simulink model "EcoSIM3_P2_C2_WIP"  (R2014b)
settings: Solver=ode1  SolverMode=SingleTasking  StartTime=0.0  StopTime=4  FixedStep=0.01  RelTol=1e-3
PostLoadFcn:
  | %, if any(exist('dsrtsu_mdlpostloadfcn', 'file') == [2, 3, 6]), try dsrtsu_mdlpostloadfcn('Execute', bdroot); catch fprintf('Error in PostLoadFcn (dsrtsu_mdlpostloadfcn) for model "%s":\n %s\n', bdroot, lasterr); end, end,
InitFcn:
  | tic
  | %Startup_EcoSIM
undefined symbols (not defined in the file or in its folder): canChannel, Controls, DriveCycles, Driver, EM_EFF_MAP, EM_PwrLoss_MAP, EngPwr, EngSpd, EngTrq, Glbl, Overwritten_Mode, Plants, Power, sigbuilder_block, Torque, Trialmap, Veh_Dynamics
libraries: simulink x135, canmsglib x113, fl_lib x104, canlib x89, nesl_utility x56, sdl_lib x29, dspsigops x6, dspswit3 x5, dspstat3 x2, commnoisgen2 x1, dspfdesign x1
(part 16 of 21)

== system EcoSIM3_P2_C2_WIP/Powertrain/Clutch_Transmission2/Trans_Plant/Plant/Subsystem/Lookup Table based Gear ==
  y12 : Inport
  y34 : Inport  Port=2
  y5R : Inport  Port=3
  Bias : Bias  Bias=-1
  Bias1 : Bias  Bias=-1
  Bias2 : Bias  Bias=-1
  Direct Lookup Table (n-D) : LookupNDDirect  NumberOfTableDimensions=3  Table=cat(3,[8 8 8; 8 5 8; 8 8 8], [8 1 8; 3 0 4; 8 2 8],[8 8 8; 8 -1 8; 8 8 8])
  Gear : Outport
  wires:
  Bias/1 -> Direct Lookup Table (n-D)/1
  Bias1/1 -> Direct Lookup Table (n-D)/2
  Bias2/1 -> Direct Lookup Table (n-D)/3
  y12/1 -> Bias/1
  Direct Lookup Table (n-D)/1 -> Gear/1
  y5R/1 -> Bias2/1
  y34/1 -> Bias1/1

== system EcoSIM3_P2_C2_WIP/Powertrain/Electric Motor / Component Model/Plant/EM_Thermal_Model/EM_Over_Temp_Fault ==
  In1 : Inport
  Bus Selector : BusSelector  OutputSignals=Temp_deg_C,EM_OverTemp_Trigger
  Switch : Switch  Criteria=u2 > Threshold  Threshold=0.5
  Out1 : Outport
  wires:
  [EM_Over_temperature_Trigger] -> Bus Selector/1
  Bus Selector/1 -> Switch/1  "<Temp_deg_C>"
  Bus Selector/2 -> Switch/2  "<EM_OverTemp_Trigger>"
  Switch/1 -> Out1/1
  In1/1 -> Switch/3

== system EcoSIM3_P2_C2_WIP/Powertrain/Electric Motor / Component Model/Plant/EM_Thermal_Model/Heat Dissipated through coolant ==
  Coolant Out Temp : Inport
  Add1 : Sum  Inputs=+-
  Coolant Heat Capacity : Gain  Gain=3148
  Coolant Flow rate lit/min : Constant  Value=4
  Coolant Inlet Temp (K) : Constant  Value=293
  Product : Product
  Simulink-PS Converter2 : nesl_utility/Simulink-PS Converter  PhysicalDomain=network_engine_domain  SubClassName=ps_input  LeftPortType=input  RightPortType=output  PseudoPeriodic=off  Frequencies=[]  NoiseDistribution=none  NoiseParameters=[]  Unit=J/s  AffineConversion=off  InputFiltering=off  SimscapeFilterOrder=1  InputFilterTimeConstant=0.001  UdotUserProvided=1
  Subtract : Gain  Gain=-1
  per sec : Gain  Gain=1/60
  Coolant Heat Gain : PMIOPort  Port=1  Side=Right
  wires:
  Product/1 -> Subtract/1  "EM_Coolant_Heat_Reject_W"
  Coolant Heat Capacity/1 -> Product/2
  Add1/1 -> Product/1
  Coolant Inlet Temp (K)/1 -> Add1/2
  Subtract/1 -> Simulink-PS Converter2/1
  Coolant Out Temp/1 -> Add1/1
  per sec/1 -> Coolant Heat Capacity/1
  Coolant Flow rate lit/min/1 -> per sec/1
  connections:
  Simulink-PS Converter2/RConn1 -- Coolant Heat Gain/RConn1

== system EcoSIM3_P2_C2_WIP/Powertrain/Electric Motor / Component Model/Plant/EM_Thermal_Model/Temp Hotspot ==
  Add1 : Sum  Inputs=+-
  Constant3 : Constant  Value=273
  Ideal Temperature Sensor1 : fl_lib/Thermal/Thermal Sensors/Ideal Temperature Sensor
  PS-Simulink Converter1 : nesl_utility/PS-Simulink Converter  PhysicalDomain=network_engine_domain  SubClassName=ps_output  LeftPortType=input  RightPortType=output  PseudoPeriodic=off  Frequencies=[]  Unit=K  AffineConversion=off
  Thermal Reference5 : fl_lib/Thermal/Thermal Elements/Thermal Reference
  Conn1 : PMIOPort  Port=1  Side=Left
  Temp C : Outport
  wires:
  Constant3/1 -> Add1/2
  PS-Simulink Converter1/1 -> Add1/1
  Add1/1 -> Temp C/1
  connections:
  Ideal Temperature Sensor1/RConn2 -- PS-Simulink Converter1/LConn1
  Thermal Reference5/LConn1 -- Ideal Temperature Sensor1/RConn1
  Ideal Temperature Sensor1/LConn1 -- Conn1/RConn1

== system EcoSIM3_P2_C2_WIP/Powertrain/Electric Motor / Component Model/Plant/EM_Thermal_Model/Temp Motor ==
  Add : Sum  Inputs=+-
  Constant2 : Constant  Value=273
  Ideal Temperature Sensor : fl_lib/Thermal/Thermal Sensors/Ideal Temperature Sensor
  PS-Simulink Converter : nesl_utility/PS-Simulink Converter  PhysicalDomain=network_engine_domain  SubClassName=ps_output  LeftPortType=input  RightPortType=output  PseudoPeriodic=off  Frequencies=[]  Unit=K  AffineConversion=off
  Thermal Reference1 : fl_lib/Thermal/Thermal Elements/Thermal Reference
  Temp in : PMIOPort  Port=1  Side=Left
  Temp K : Outport
  Temp C : Outport  Port=2
  wires:
  PS-Simulink Converter/1 -> Temp K/1, Add/1
  Add/1 -> Temp C/1
  Constant2/1 -> Add/2
  connections:
  Ideal Temperature Sensor/RConn2 -- PS-Simulink Converter/LConn1
  Thermal Reference1/LConn1 -- Ideal Temperature Sensor/RConn1
  Temp in/RConn1 -- Ideal Temperature Sensor/LConn1

== system EcoSIM3_P2_C2_WIP/Powertrain/Electric Motor / Component Model/Sensors/Sensors/Sensor lag ==
  i : Inport
  1st Order LPF of 1ms in Discrete Form : DiscreteTransferFcn  Numerator=[0.6321]  Denominator=[1 -0.3679]
  o : Outport
  wires:
  i/1 -> 1st Order LPF of 1ms in Discrete Form/1
  1st Order LPF of 1ms in Discrete Form/1 -> o/1

== system EcoSIM3_P2_C2_WIP/Powertrain/Electric Motor / Component Model/Sensors/Sensors/Sensor lag1 ==
  i : Inport
  1st Order LPF of 1ms in Discrete Form : DiscreteTransferFcn  Numerator=[0.6321]  Denominator=[1 -0.3679]
  o : Outport
  wires:
  i/1 -> 1st Order LPF of 1ms in Discrete Form/1
  1st Order LPF of 1ms in Discrete Form/1 -> o/1

== system EcoSIM3_P2_C2_WIP/Powertrain/Electric Motor /Soft ECU/Algorithm/Normal Operation/EEPROM Parameters1 ==
  note: Key Switch Mode Always set to 0. Refer to RMS Hardware user manual
  Bus Creator : BusCreator  Inputs=3
  KeySwMode : Constant  Value=0
  Motor_MaxSpeed : Constant  Value=max(Plants.EM.Mdl.Plant.max_min_w)
  POST_Fault : Constant  Value=0
  EEPROM param : Outport
  wires:
  Motor_MaxSpeed/1 -> Bus Creator/1  "Motor_MaxSpeed"
  KeySwMode/1 -> Bus Creator/2  "KeySwMode"
  Bus Creator/1 -> EEPROM param/1
  POST_Fault/1 -> Bus Creator/3  "POST_Fault"

== system EcoSIM3_P2_C2_WIP/Powertrain/Electric Motor /Soft ECU/Algorithm/Startup_Shutdown/EEPROM Parameters ==
  note: Key Switch Mode Always set to 0. Refer to RMS Hardware user manual
  Bus Creator : BusCreator  Inputs=3
  KeySwMode : Constant  Value=0
  Motor_MaxSpeed : Constant  Value=max(Plants.EM.Mdl.Plant.max_min_w)
  POST_Fault : Constant  Value=0
  EEPROM param : Outport
  wires:
  Motor_MaxSpeed/1 -> Bus Creator/1  "Motor_MaxSpeed"
  KeySwMode/1 -> Bus Creator/2  "KeySwMode"
  Bus Creator/1 -> EEPROM param/1
  POST_Fault/1 -> Bus Creator/3  "POST_Fault"

== system EcoSIM3_P2_C2_WIP/Powertrain/Electric Motor /Soft ECU/Algorithm/Startup_Shutdown/Subsystem ==
  Dir_In : Inport
  VSM_In : Inport  Port=2
  Bus Selector3 : BusSelector  OutputSignals=vsm_state_value,vsm_state_trigger
  Compare To Constant : simulink/Logic and Bit Operations/Compare To Constant  relop===  const=6  OutDataTypeStr=boolean
  Data Type Conversion : DataTypeConversion
  Product : Product
  Switch : Switch  Criteria=u2 > Threshold  Threshold=0.5
  Dir : Outport
  VSM : Outport  Port=2
  wires:
  [VSM_State_Trigger] -> Bus Selector3/1
  VSM_In/1 -> Switch/3
  Bus Selector3/2 -> Switch/2  "<vsm_state_trigger>"
  Bus Selector3/1 -> Switch/1  "<vsm_state_value>"
  Switch/1 -> Compare To Constant/1, VSM/1  "VSM_State"
  Product/1 -> Data Type Conversion/1
  Compare To Constant/1 -> Product/1
  Dir_In/1 -> Product/2
  Data Type Conversion/1 -> Dir/1  "Direction_Command_Feedback"

== system EcoSIM3_P2_C2_WIP/Powertrain/Electric Motor /Soft ECU/Algorithm/Startup_Shutdown/Temperature Values Dummy ==
  FromPlant : Inport
  Bus Creator : BusCreator  Inputs=6
  Control_Board_Temperature : Constant  Value=25
  ESS_Over_Temp_Fault : Subsystem
  Gain : Gain
  Gate_Driver_Board : Constant  Value=25
  Module_A : Constant  Value=25
  Module_B : Constant  Value=25
  Module_C : Constant  Value=25
  TempValues : Outport
  wires:
  ESS_Over_Temp_Fault/1(Out1) -> Bus Creator/1  "Module_A"
  Bus Creator/1 -> TempValues/1
  Module_B/1 -> Bus Creator/2  "Module_B"
  Module_C/1 -> Bus Creator/3  "Module_C"
  Gate_Driver_Board/1 -> Bus Creator/4  "Gate_Driver_Board"
  Control_Board_Temperature/1 -> Bus Creator/5  "Control_Board_Temperature"
  FromPlant/1 -> Gain/1
  Gain/1 -> Bus Creator/6  "Motor_Temperature"
  Module_A/1 -> ESS_Over_Temp_Fault/1(In1)

== system EcoSIM3_P2_C2_WIP/Powertrain/Electrical Storage System/ ESS Model/Plant/Electrical Plant Model/Current Calculation (Per Cell) ==
  note: 3
  P_in [W] : Inport
  Batt_volt [V] : Inport  Port=2
  Battery capacity1 : Gain  Gain=1/(Plants.ESS.Mdl.Plant.EPM.Curr_Calc.P)
  Divide : Product  Inputs=*/
  Batt_Current [A] : Outport
  Cell_Current [A] : Outport  Port=2
  wires:
  P_in [W]/1 -> Divide/1
  Divide/1 -> Batt_Current [A]/1, Battery capacity1/1  "Batt_Current_A"
  Batt_volt [V]/1 -> Divide/2
  Battery capacity1/1 -> Cell_Current [A]/1  "Batt_Cell_Current_A]"

== system EcoSIM3_P2_C2_WIP/Powertrain/Electrical Storage System/ ESS Model/Plant/Electrical Plant Model/Heat Calculation ==
  note: 315
  Cell_Current [A] : Inport
  R_cell [Ohms] : Inport  Port=2
  Fcn : Fcn  Expr=u^2
  Gain : Gain
  Heat input for pack : Gain  Gain=Plants.ESS.Mdl.Plant.EPM.Heat_Calc.N
  Product : Product
  Terminator : Terminator
  Batt_Heat [W] : Outport
  wires:
  Fcn/1 -> Product/1
  R_cell [Ohms]/1 -> Gain/1, Product/2
  Product/1 -> Heat input for pack/1
  Heat input for pack/1 -> Batt_Heat [W]/1  "Batt_Heat_W"
  Cell_Current [A]/1 -> Fcn/1
  Gain/1 -> Terminator/1  "R_cell"

== system EcoSIM3_P2_C2_WIP/Powertrain/Electrical Storage System/ ESS Model/Plant/Electrical Plant Model/OCV Estimation ==
  note: if I>0 --> DISCHARGE
  note: if I<0 --> CHARGE
  SOC [%] : Inport
  Cell_Current [A] : Inport  Port=2
  Charge : Subsystem
  Discharge : Subsystem
  Switch CHARGE OR DISCHARGE : Switch  Criteria=u2 > Threshold
  OCV [V] : Outport
  wires:
  Discharge/1(OCV [V]) -> Switch CHARGE OR DISCHARGE/1
  Charge/1(OCV [V]) -> Switch CHARGE OR DISCHARGE/3
  Cell_Current [A]/1 -> Switch CHARGE OR DISCHARGE/2
  Switch CHARGE OR DISCHARGE/1 -> OCV [V]/1  "Batt_Cell_OCV_V"
  SOC [%]/1 -> Discharge/1(SOC [%]), Charge/1(SOC [%])

== system EcoSIM3_P2_C2_WIP/Powertrain/Electrical Storage System/ ESS Model/Plant/Electrical Plant Model/Resistance Estimation (Per Cell)  ==
  note: if I>0 --> DISCHARGE
  note: if I<0 --> CHARGE
  Cell_Current [A] : Inport
  Cell_Temp [C] : Inport  Port=2
  SOC [%] : Inport  Port=3
  Charge : Subsystem
  Discharge : Subsystem
  Switch CHARGE OR DISCHARGE : Switch  Criteria=u2 > Threshold
  R_cell [Ohms] : Outport
  wires:
  Discharge/1(R_cell [Ohms]) -> Switch CHARGE OR DISCHARGE/1
  Charge/1(R_cell [Ohms]) -> Switch CHARGE OR DISCHARGE/3
  Cell_Current [A]/1 -> Switch CHARGE OR DISCHARGE/2
  Switch CHARGE OR DISCHARGE/1 -> R_cell [Ohms]/1  "Batt_Cell_Resistance_Ohms"
  Cell_Temp [C]/1 -> Charge/1(Temp [C]), Discharge/1(Temp [C])
  SOC [%]/1 -> Discharge/2(SOC [%]), Charge/2(SOC [%])

== system EcoSIM3_P2_C2_WIP/Powertrain/Electrical Storage System/ ESS Model/Plant/Electrical Plant Model/SOC Estimation (Per Cell) ==
  note: 1/Gain2
  note: Gain2
  note: (19.6*3600*1000)/100
  note: -1 What is this?
  P_in [W] : Inport
  A.h to A.sec1 : Gain  Gain=1/Plants.ESS.Mdl.Plant.EPM.SOC_Est.Gain2
  Bus Selector : BusSelector  OutputSignals=Init_SOC_percent
  Gain1 : Gain  Gain=Plants.ESS.Mdl.Plant.EPM.SOC_Est.Gain1
  Integrator Limited : Integrator  InitialConditionSource=external  InitialCondition=19.6*3600*1000  LimitOutput=on  UpperSaturationLimit=19.6*3600*1000  LowerSaturationLimit=0
  SOC : Gain  Gain=Plants.ESS.Mdl.Plant.EPM.SOC_Est.Gain2
  SOC [%] : Outport
  wires:
  Integrator Limited/1 -> A.h to A.sec1/1
  Gain1/1 -> Integrator Limited/1
  P_in [W]/1 -> Gain1/1
  A.h to A.sec1/1 -> SOC [%]/1  "Batt_SOC_percent"
  SOC/1 -> Integrator Limited/2
  [Simulation_Parameters] -> Bus Selector/1
  Bus Selector/1 -> SOC/1  "<Init_SOC_percent>"

== system EcoSIM3_P2_C2_WIP/Powertrain/Electrical Storage System/ ESS Model/Plant/Electrical Plant Model/Terminal Voltage Calculation ==
  note: 105
  R_cell [Ohms] : Inport
  OCV [V] : Inport  Port=2
  Cell_Current [A] : Inport  Port=3
  Add : Sum  Inputs=+-
  Pack voltage : Gain  Gain=Plants.ESS.Mdl.Plant.EPM.Term_V_calc.S
  Product1 : Product
  Batt_Volt [V] : Outport
  wires:
  Product1/1 -> Add/2
  Add/1 -> Pack voltage/1
  OCV [V]/1 -> Add/1
  Cell_Current [A]/1 -> Product1/1
  R_cell [Ohms]/1 -> Product1/2
  Pack voltage/1 -> Batt_Volt [V]/1  "Batt_Voltage_V"

== system EcoSIM3_P2_C2_WIP/Powertrain/Electrical Storage System/ ESS Model/Plant/Power Calculation/Avg Power Calculation ==
  note: EM+BAS+Accessories
  Input_Crnt [A] : Inport
  Batt_volt_1 [V] : Inport  Port=2
  Component_Power_Watts : Inport  Port=3
  " " : Sum  SaturateOnIntegerOverflow=on  InputSameDT=on  OutDataTypeStr=Inherit: Same as first input
  Divide1 : Product  Inputs=**
  P_in [W] : Outport
  wires:
  Input_Crnt [A]/1 -> Divide1/1
  Batt_volt_1 [V]/1 -> Divide1/2
  Divide1/1 -> " "/1
  " "/1 -> P_in [W]/1  "Batt_P_In_W"
  Component_Power_Watts/1 -> " "/2

== system EcoSIM3_P2_C2_WIP/Powertrain/Electrical Storage System/ ESS Model/Plant/Thermal Model/ESS_Over_Temp_Fault ==
  In1 : Inport
  Add : Sum
  Bus Selector : BusSelector  OutputSignals=ESS_OverTemp_Trigger
  Integrator : Integrator  ExternalReset=rising
  Switch : Switch  Commented=on  Criteria=u2 > Threshold  Threshold=0.5
  Out1 : Outport
  wires:
  [ESS_Over_temperature_Trigger] -> Bus Selector/1
  Add/1 -> Out1/1
  In1/1 -> Add/2
  Bus Selector/1 -> Integrator/1, Integrator/2  "<ESS_OverTemp_Trigger>"
  Integrator/1 -> Add/1

== system EcoSIM3_P2_C2_WIP/Powertrain/Electrical Storage System/Soft ECU/Algorithm/Current Buffer/Charge Buffer ==
  note: Allow only negativd (charging) currents
  Current : Inport
  Gain : Gain  Gain=-1
  Moderator-Opposer : Subsystem
  RollingAverage : Subsystem
  Saturation6 : Saturate  UpperLimit=0  LowerLimit=-inf
  Terminator : Terminator
  Buffer : Outport
  wires:
  Moderator-Opposer/1(Buffer) -> Buffer/1
  Current/1 -> Saturation6/1
  Saturation6/1 -> Gain/1
  RollingAverage/1(Buffer) -> Terminator/1
  Gain/1 -> RollingAverage/1(Batt_Current), Moderator-Opposer/1(Current)

== system EcoSIM3_P2_C2_WIP/Powertrain/Electrical Storage System/Soft ECU/Algorithm/Current Buffer/Current based EPO ==
  dis_max : Inport
  i_bat : Inport  Port=2
  Add : Sum  Inputs=+-
  Compare To Constant : simulink/Logic and Bit Operations/Compare To Constant  relop=>=  const=10000  OutDataTypeStr=boolean
  Gain : Gain  Gain=-1
  Integrator : Integrator  ExternalReset=rising
  Math Function : Math  Operator=square  SaturateOnIntegerOverflow=on
  Saturation : Saturate  UpperLimit=inf  LowerLimit=0
  Sign : Signum
  epo_req : Outport
  wires:
  Sign/1 -> Gain/1
  Saturation/1 -> Math Function/1
  Integrator/1 -> Compare To Constant/1
  Add/1 -> Sign/1, Saturation/1
  Math Function/1 -> Integrator/1
  Gain/1 -> Integrator/2
  Compare To Constant/1 -> epo_req/1
  dis_max/1 -> Add/2
  i_bat/1 -> Add/1

== system EcoSIM3_P2_C2_WIP/Powertrain/Electrical Storage System/Soft ECU/Algorithm/Current Buffer/Discharge Buffer ==
  Current : Inport
  Constant : Constant  Value=408
  Constant1 : Constant  Value=120
  Moderator-Opposer : Subsystem
  RollingAverage : Subsystem
  Saturation : Saturate  UpperLimit=inf  LowerLimit=0
  Switch : Switch  Criteria=u2 > Threshold
  Terminator : Terminator
  Buffer : Outport
  dis_max : Outport  Port=2
  wires:
  Saturation/1 -> RollingAverage/1(Batt_Current), Moderator-Opposer/1(Current)
  Current/1 -> Saturation/1
  Moderator-Opposer/1(Buffer) -> Switch/2, Buffer/1
  RollingAverage/1(Buffer) -> Terminator/1
  Constant/1 -> Switch/1
  Constant1/1 -> Switch/3
  Switch/1 -> dis_max/1

== system EcoSIM3_P2_C2_WIP/Powertrain/Engine/Soft ECU/Algorithm/TorqueRegulation/Enabled Subsystem ==
  Red_Line_Speed : Inport
  Engine_Speed [rad/s] : Inport  Port=2
  Enable : EnablePort
  Compare To Zero1 : simulink/Logic and Bit Operations/Compare To Zero  relop===  OutDataTypeStr=boolean  ZeroCross=off
  Delay : Subsystem
  I : Constant  Value=0.1
  Integrator1 : Integrator  ExternalReset=level
  P : Constant  Value=120
  Product3 : Product  RndMeth=Zero
  Product4 : Product  RndMeth=Zero
  Sum3 : Sum  Inputs=|-+  SaturateOnIntegerOverflow=on  InputSameDT=on  OutDataTypeStr=Inherit: Same as first input
  Sum4 : Sum  SaturateOnIntegerOverflow=on  InputSameDT=on  OutDataTypeStr=Inherit: Same as first input
  Sum5 : Sum  Inputs=|+-  SaturateOnIntegerOverflow=on  InputSameDT=on  OutDataTypeStr=Inherit: Same as first input
  "Torque Command " : Outport
  wires:
  I/1 -> Product3/2
  Sum5/1 -> Product4/2
  Delay/1(Pre_Engine_Speed_Rad_per_sec) -> Sum3/2
  Red_Line_Speed/1 -> Sum5/1, Delay/1(Engine_Speed_Rad_per_sec)
  P/1 -> Product4/1
  Sum3/1 -> Integrator1/1
  Integrator1/1 -> Product3/1
  Product4/1 -> Sum4/1
  Product3/1 -> Sum4/2
  Compare To Zero1/1 -> Integrator1/2
  Engine_Speed [rad/s]/1 -> Sum5/2, Compare To Zero1/1, Sum3/1
  Sum4/1 -> "Torque Command "/1

== system EcoSIM3_P2_C2_WIP/Powertrain/Engine/Soft ECU/Algorithm/TorqueRegulation/Enabled Subsystem1 ==
  Idle_Speed : Inport
  Engine_Speed [rad/s] : Inport  Port=2
  Enable : EnablePort
  Compare To Zero1 : simulink/Logic and Bit Operations/Compare To Zero  relop===  OutDataTypeStr=boolean  ZeroCross=off
  Delay : Subsystem
  I : Constant  Value=0.1
  Integrator1 : Integrator  ExternalReset=level
  P : Constant  Value=120
  Product3 : Product  RndMeth=Zero
  Product4 : Product  RndMeth=Zero
  Sum3 : Sum  Inputs=|-+  SaturateOnIntegerOverflow=on  InputSameDT=on  OutDataTypeStr=Inherit: Same as first input
  Sum4 : Sum  SaturateOnIntegerOverflow=on  InputSameDT=on  OutDataTypeStr=Inherit: Same as first input
  Sum5 : Sum  Inputs=|+-  SaturateOnIntegerOverflow=on  InputSameDT=on  OutDataTypeStr=Inherit: Same as first input
  "Torque Command " : Outport
  wires:
  Sum4/1 -> "Torque Command "/1
  Engine_Speed [rad/s]/1 -> Sum3/1, Compare To Zero1/1, Sum5/2
  Compare To Zero1/1 -> Integrator1/2
  Product3/1 -> Sum4/2
  Product4/1 -> Sum4/1
  Integrator1/1 -> Product3/1
  Sum3/1 -> Integrator1/1
  P/1 -> Product4/1
  Idle_Speed/1 -> Delay/1(Engine_Speed_Rad_per_sec), Sum5/1
  Delay/1(Pre_Engine_Speed_Rad_per_sec) -> Sum3/2
  Sum5/1 -> Product4/2
  I/1 -> Product3/2

== system EcoSIM3_P2_C2_WIP/Powertrain/Engine/Soft ECU/Algorithm/TorqueRegulation/Enabled Subsystem2 ==
  Torque_Cmd_Nm : Inport
  Engine Speed [rad/s] : Inport  Port=2
  Enable : EnablePort
  Constant : Constant  Value=0
  Max Torque : Lookup_n-D  NumberOfTableDimensions=1  BreakpointsForDimension1=Plants.ICE.Mdl.Plant.Max_Trq.w  Table=Plants.ICE.Mdl.Plant.Max_Trq.Trq  InternalRulePriority=Speed  RndMeth=Simplest  InputSameDT=on
  Saturation Dynamic : simulink/Discontinuities/Saturation Dynamic  OutMin=[]  OutMax=[]  OutDataTypeStr=Inherit: Same as second input  OutDataType=fixdt(1, 16)  OutScaling=2^-10  DoSatur=off
  "Torque Command " : Outport
  wires:
  Torque_Cmd_Nm/1 -> Saturation Dynamic/2
  Engine Speed [rad/s]/1 -> Max Torque/1
  Max Torque/1 -> Saturation Dynamic/1
  Constant/1 -> Saturation Dynamic/3
  Saturation Dynamic/1 -> "Torque Command "/1

== system EcoSIM3_P2_C2_WIP/Powertrain/Engine/Soft ECU/Algorithm/TorqueRegulation/Subsystem ==
  Engine_Speed : Inport
  ECM_Powerup : Inport  Port=2
  Torque_Request : Inport  Port=3
  ISP_R : Inport  Port=4
  PCM_Wake : Inport  Port=5
  Chart : Stateflow chart  TreatAsAtomicUnit=on
  Constant : Constant  Value=Plants.ICE.Mdl.Plant.red_line_w
  Constant1 : Constant  Value=0.9722*Plants.ICE.Mdl.Plant.idle_w
  Constant2 : Constant  Value=0.9583*Plants.ICE.Mdl.Plant.idle_w
  IC : InitialCondition
  Memory : Memory  X0=1
  Mode : Outport
  Torque_Cmd : Outport  Port=2
  wires:
  Chart/2(Mode) -> Memory/1
  ECM_Powerup/1 -> Chart/2(ECM_Powerup)
  Torque_Request/1 -> Chart/3(Torque_Request)
  Constant/1 -> Chart/6(Max_Speed)
  PCM_Wake/1 -> Chart/4(PCM_Wake)
  Constant1/1 -> Chart/7(Upper_Idle_Speed_Bound)
  Constant2/1 -> Chart/8(Lower_Idle_Speed_Bound)
  ISP_R/1 -> Chart/5(ISP_R)
  Engine_Speed/1 -> Chart/1(Engine_Speed)
  Chart/1(Torque_Cmd) -> Torque_Cmd/1
  Memory/1 -> Mode/1

== system EcoSIM3_P2_C2_WIP/Powertrain/Soft_ECUs_IO/VNT Kvaser/CANTx/EM/M160_Temperature_Set_1 ==
  EM : Inport
  Bus Selector5 : BusSelector  OutputSignals=M160_Temperature_Set_1.Module_A,M160_Temperature_Set_1.Module_B,M160_Temperature_Set_1.Module_C,M160_Temperature_Set_1.Gate_Driver_Board
  CAN Pack3 : canmsglib/CAN Pack  CANdbFile=C:\Users\EcoCAR_HIL\Documents\Khanna\EcoSIM3_P1_0_PHEV_TCU\Final_DBC\20150828 RMS PM CAN DB.dbc  MsgList=M160_Temperature_Set_1  MsgName=M160_Temperature_Set_1  MsgIDType=Standard (11-bit identifier)  MsgIdentifier=160  MsgLength=8  SignalInfo=D1_Module_A$0$16$1$1$1$0$1.000000e-01$0$-3.276800e+03$3.276700e+03$#D2_Module_B$16$16$1$1$1$0$1.000000e-01$0$-3.276800e+03$3.276700e+03$#D3_Module_C$32$16$1$1$1$0$1.000000e-01$0$-3.276800e+03$3.276700e+03$#D4_Gate_Driver_Board$48$16$1$1$1$0$1.000000e-01$0$-3.276800e+03$3.276700e+03$#  NSignals=4  StartBits=str2num('[int32(0);int32(16);int32(32);int32(48)]')  SignalSizes=str2num('[int32(16);int32(16);int32(16);int32(16)]')  ByteOrders=str2num('[int32(1);int32(1);int32(1);int32(1)]')  DataTypes=str2num('[int32(1);int32(1);int32(1);int32(1)]')  MultiplexTypes=str2num('[int32(1);int32(1);int32(1);int32(1)]')  MultiplexValues=str2num('[double(0);double(0);double(0);double(0)]')  Factors=str2num('[double(1.000000e-01);double(1.000000e-01);double(1.000000e-01);double(1.000000e-01)]')  Offsets=str2num('[double(0);double(0);double(0);double(0)]')  Minimums=str2num('[double(-3.276800e+03);double(-3.276800e+03);double(-3.276800e+03);double(-3.276800e+03)]')  Maximums=str2num('[double(3.276700e+03);double(3.276700e+03);double(3.276700e+03);double(3.276700e+03)]')  Remote=off
      settings: DataFormat=CANdb specified signals
  CAN Transmit1 : canlib/CAN Transmit  BlockHandle=2890.0023  DeviceMenu=Kvaser Virtual 1 (Channel 2)  Device=Kvaser Virtual 1 (Channel 2)  ObjConstructor=canChannel('Kvaser', 'Virtual 1', 2)  EnablePeriodicTransmit=off  MessagePeriod=1.000
  Rate Transition{,1..3} (4 alike) : RateTransition
  wires:
  Bus Selector5/2 -> Rate Transition3/1  "<Module_B>"
  Bus Selector5/4 -> Rate Transition1/1  "<Gate_Driver_Board>"
  Bus Selector5/1 -> Rate Transition/1  "<Module_A>"
  Bus Selector5/3 -> Rate Transition2/1  "<Module_C>"
  EM/1 -> Bus Selector5/1
  Rate Transition/1 -> CAN Pack3/1
  Rate Transition1/1 -> CAN Pack3/4
  Rate Transition2/1 -> CAN Pack3/3
  Rate Transition3/1 -> CAN Pack3/2
  CAN Pack3/1 -> CAN Transmit1/1

== system EcoSIM3_P2_C2_WIP/Powertrain/Soft_ECUs_IO/VNT Kvaser/CANTx/EM/M161_Temperature_Set_2 ==
  EM : Inport
  Bus Selector6 : BusSelector  OutputSignals=M161_Temperature_Set_2.Control_Board_Temperature
  CAN Pack5 : canmsglib/CAN Pack  CANdbFile=C:\Users\EcoCAR_HIL\Documents\Khanna\EcoSIM3_P1_0_PHEV_TCU\Final_DBC\20150828 RMS PM CAN DB.dbc  MsgList=M161_Temperature_Set_2  MsgName=M161_Temperature_Set_2  MsgIDType=Standard (11-bit identifier)  MsgIdentifier=161  MsgLength=8  SignalInfo=D1_Control_Board_Temperature$0$16$1$1$1$0$1.000000e-01$0$-3.276800e+03$3.276700e+03$#D2_RTD1_Temperature$16$16$1$1$1$0$1.000000e-01$0$-3.276800e+03$3.276700e+03$#D3_RTD2_Temperature$32$16$1$1$1$0$1.000000e-01$0$-3.276800e+03$3.276700e+03$#D4_RTD3_Temperature$48$16$1$1$1$0$1.000000e-01$0$-3.276800e+03$3.276700e+03$#  NSignals=4  StartBits=str2num('[int32(0);int32(16);int32(32);int32(48)]')  SignalSizes=str2num('[int32(16);int32(16);int32(16);int32(16)]')  ByteOrders=str2num('[int32(1);int32(1);int32(1);int32(1)]')  DataTypes=str2num('[int32(1);int32(1);int32(1);int32(1)]')  MultiplexTypes=str2num('[int32(1);int32(1);int32(1);int32(1)]')  MultiplexValues=str2num('[double(0);double(0);double(0);double(0)]')  Factors=str2num('[double(1.000000e-01);double(1.000000e-01);double(1.000000e-01);double(1.000000e-01)]')  Offsets=str2num('[double(0);double(0);double(0);double(0)]')  Minimums=str2num('[double(-3.276800e+03);double(-3.276800e+03);double(-3.276800e+03);double(-3.276800e+03)]')  Maximums=str2num('[double(3.276700e+03);double(3.276700e+03);double(3.276700e+03);double(3.276700e+03)]')  Remote=off
      settings: DataFormat=CANdb specified signals
  CAN Transmit1 : canlib/CAN Transmit  BlockHandle=2909.0023  DeviceMenu=Kvaser Virtual 1 (Channel 2)  Device=Kvaser Virtual 1 (Channel 2)  ObjConstructor=canChannel('Kvaser', 'Virtual 1', 2)  EnablePeriodicTransmit=off  MessagePeriod=1.000
  Ground5 : Ground
  Rate Transition : RateTransition
  wires:
  Bus Selector6/1 -> Rate Transition/1  "<Control_Board_Temperature>"
  Ground5/1 -> CAN Pack5/3, CAN Pack5/2, CAN Pack5/4
  EM/1 -> Bus Selector6/1
  Rate Transition/1 -> CAN Pack5/1
  CAN Pack5/1 -> CAN Transmit1/1

== system EcoSIM3_P2_C2_WIP/Powertrain/Soft_ECUs_IO/VNT Kvaser/CANTx/EM/M162_Temperature_Set_3 ==
  EM : Inport
  Bus Selector7 : BusSelector  OutputSignals=M162_Temperature_Set_3.Motor_Temperature
  CAN Pack6 : canmsglib/CAN Pack  CANdbFile=C:\Users\EcoCAR_HIL\Documents\Khanna\EcoSIM3_P1_0_PHEV_TCU\Final_DBC\20150828 RMS PM CAN DB.dbc  MsgList=M162_Temperature_Set_3  MsgName=M162_Temperature_Set_3  MsgIDType=Standard (11-bit identifier)  MsgIdentifier=162  MsgLength=8  SignalInfo=D1_RTD4_Temperature$0$16$1$1$1$0$1.000000e-01$0$-3.276800e+03$3.276700e+03$#D2_RTD5_Temperature$16$16$1$1$1$0$1.000000e-01$0$-3.276800e+03$3.276700e+03$#D3_Motor_Temperature$32$16$1$1$1$0$1.000000e-01$0$-3.276800e+03$3.276700e+03$#D4_Torque_Shudder$48$16$1$1$1$0$1.000000e-01$0$-3.276800e+03$3.276700e+03$#  NSignals=4  StartBits=str2num('[int32(0);int32(16);int32(32);int32(48)]')  SignalSizes=str2num('[int32(16);int32(16);int32(16);int32(16)]')  ByteOrders=str2num('[int32(1);int32(1);int32(1);int32(1)]')  DataTypes=str2num('[int32(1);int32(1);int32(1);int32(1)]')  MultiplexTypes=str2num('[int32(1);int32(1);int32(1);int32(1)]')  MultiplexValues=str2num('[double(0);double(0);double(0);double(0)]')  Factors=str2num('[double(1.000000e-01);double(1.000000e-01);double(1.000000e-01);double(1.000000e-01)]')  Offsets=str2num('[double(0);double(0);double(0);double(0)]')  Minimums=str2num('[double(-3.276800e+03);double(-3.276800e+03);double(-3.276800e+03);double(-3.276800e+03)]')  Maximums=str2num('[double(3.276700e+03);double(3.276700e+03);double(3.276700e+03);double(3.276700e+03)]')  Remote=off
      settings: DataFormat=CANdb specified signals
  CAN Transmit1 : canlib/CAN Transmit  BlockHandle=2924.0023  DeviceMenu=Kvaser Virtual 1 (Channel 2)  Device=Kvaser Virtual 1 (Channel 2)  ObjConstructor=canChannel('Kvaser', 'Virtual 1', 2)  EnablePeriodicTransmit=off  MessagePeriod=1.000
  Ground6 : Ground
  Rate Transition : RateTransition
  wires:
  Ground6/1 -> CAN Pack6/1, CAN Pack6/2, CAN Pack6/4
  Bus Selector7/1 -> Rate Transition/1  "<Motor_Temperature>"
  EM/1 -> Bus Selector7/1
  Rate Transition/1 -> CAN Pack6/3
  CAN Pack6/1 -> CAN Transmit1/1

== system EcoSIM3_P2_C2_WIP/Powertrain/Soft_ECUs_IO/VNT Kvaser/CANTx/EM/M165_Motor_Position_Info ==
  EM : Inport
  Bus Selector1 : BusSelector  OutputSignals=M165_Motor_Position_Info.Motor_Speed
  CAN Pack1 : canmsglib/CAN Pack  CANdbFile=C:\Users\EcoCAR_HIL\Documents\Khanna\EcoSIM3_P1_0_PHEV_TCU\Final_DBC\20150828 RMS PM CAN DB.dbc  MsgList=M165_Motor_Position_Info  MsgName=M165_Motor_Position_Info  MsgIDType=Standard (11-bit identifier)  MsgIdentifier=165  MsgLength=8  SignalInfo=D1_Motor_Angle_Electrical$0$16$1$2$1$0$1.000000e-01$0$0$6.553500e+03$#D2_Motor_Speed$16$16$1$1$1$0$1$0$-32768$32767$#D3_Electrical_Output_Frequency$32$16$1$1$1$0$1.000000e-01$0$-3.276800e+03$3.276700e+03$#D4_Delta_Resolver_Filtered$48$16$1$1$1$0$1.000000e-01$0$-3.276800e+03$3.276700e+03$#  NSignals=4  StartBits=str2num('[int32(0);int32(16);int32(32);int32(48)]')  SignalSizes=str2num('[int32(16);int32(16);int32(16);int32(16)]')  ByteOrders=str2num('[int32(1);int32(1);int32(1);int32(1)]')  DataTypes=str2num('[int32(2);int32(1);int32(1);int32(1)]')  MultiplexTypes=str2num('[int32(1);int32(1);int32(1);int32(1)]')  MultiplexValues=str2num('[double(0);double(0);double(0);double(0)]')  Factors=str2num('[double(1.000000e-01);double(1);double(1.000000e-01);double(1.000000e-01)]')  Offsets=str2num('[double(0);double(0);double(0);double(0)]')  Minimums=str2num('[double(0);double(-32768);double(-3.276800e+03);double(-3.276800e+03)]')  Maximums=str2num('[double(6.553500e+03);double(32767);double(3.276700e+03);double(3.276700e+03)]')  Remote=off
      settings: DataFormat=CANdb specified signals
  CAN Transmit1 : canlib/CAN Transmit  BlockHandle=2940.0023  DeviceMenu=Kvaser Virtual 1 (Channel 2)  Device=Kvaser Virtual 1 (Channel 2)  ObjConstructor=canChannel('Kvaser', 'Virtual 1', 2)  EnablePeriodicTransmit=off  MessagePeriod=1.000
  Ground1 : Ground
  Rate Transition : RateTransition
  wires:
  Bus Selector1/1 -> Rate Transition/1  "<Motor_Speed>"
  Ground1/1 -> CAN Pack1/1, CAN Pack1/3, CAN Pack1/4
  EM/1 -> Bus Selector1/1
  Rate Transition/1 -> CAN Pack1/2
  CAN Pack1/1 -> CAN Transmit1/1

== system EcoSIM3_P2_C2_WIP/Powertrain/Soft_ECUs_IO/VNT Kvaser/CANTx/EM/M170_Internal_States ==
  EM : Inport
  Bus Selector3 : BusSelector  OutputSignals=M170_Internal_States.VSM_State,M170_Internal_States.Inverter_Enable_Lockout
  CAN Pack4 : canmsglib/CAN Pack  CANdbFile=C:\Users\EcoCAR_HIL\Documents\Khanna\EcoSIM3_P1_0_PHEV_TCU\Final_DBC\20150828 RMS PM CAN DB.dbc  MsgList=M170_Internal_States  MsgName=M170_Internal_States  MsgIDType=Standard (11-bit identifier)  MsgIdentifier=170  MsgLength=8  SignalInfo=D1_VSM_State$0$16$1$2$1$0$1$0$0$15$#D2_Inverter_State$16$8$1$2$1$0$1$0$0$255$#D3_Relay_1_Status$24$1$1$2$1$0$1$0$0$1$#D3_Relay_2_Status$25$1$1$2$1$0$1$0$0$1$#D3_Relay_3_Status$26$1$1$2$1$0$1$0$0$1$#D3_Relay_4_Status$27$1$1$2$1$0$1$0$0$1$#D3_Relay_5_Status$28$1$1$2$1$0$1$0$-Inf$Inf$#D3_Relay_6_Status$29$1$1$2$1$0$1$0$-Inf$Inf$#D4_Inverter_Discharge_State$37$3$1$2$1$0$1$0$0$7$#D4_Inverter_Run_Mode$32$1$1$2$1$0$1$0$0$1$#D5_Inverter_Command_Mode$40$1$1$2$1$0$1$0$0$1$#D6_Inverter_Enable_Lockout$55$1$1$2$1$0$1$0$0$1$#D6_Inverter_Enable_State$48$1$1$2$1$0$1$0$0$1$#D7_Direction_Command$56$8$1$2$1$0$1$0$0$1$#  NSignals=14  StartBits=str2num('[int32(0);int32(16);int32(24);int32(25);int32(26);int32(27);int32(28);int32(29);int32(37);int32(32);int32(40);int32(55);int32(48);int32(56)]')  SignalSizes=str2num('[int32(16);int32(8);int32(1);int32(1);int32(1);int32(1);int32(1);int32(1);int32(3);int32(1);int32(1);int32(1);int32(1);int32(8)]')  ByteOrders=str2num('[int32(1);int32(1);int32(1);int32(1);int32(1);int32(1);int32(1);int32(1);int32(1);int32(1);int32(1);int32(1);int32(1);int32(1)]')  DataTypes=str2num('[int32(2);int32(2);int32(2);int32(2);int32(2);int32(2);int32(2);int32(2);int32(2);int32(2);int32(2);int32(2);int32(2);int32(2)]')  MultiplexTypes=str2num('[int32(1);int32(1);int32(1);int32(1);int32(1);int32(1);int32(1);int32(1);int32(1);int32(1);int32(1);int32(1);int32(1);int32(1)]')  MultiplexValues=str2num('[double(0);double(0);double(0);double(0);double(0);double(0);double(0);double(0);double(0);double(0);double(0);double(0);double(0);double(0)]')  Factors=str2num('[double(1);double(1);double(1);double(1);double(1);double(1);double(1);double(1);double(1);double(1);double(1);double(1);double(1);double(1)]')  Offsets=str2num('[double(0);double(0);double(0);double(0);double(0);double(0);double(0);double(0);double(0);double(0);double(0);double(0);double(0);double(0)]')  Minimums=str2num('[double(0);double(0);double(0);double(0);double(0);double(0);double(-Inf);double(-Inf);double(0);double(0);double(0);double(0);double(0);double(0)]')  Maximums=str2num('[double(15);double(255);double(1);double(1);double(1);double(1);double(Inf);double(Inf);double(7);double(1);double(1);double(1);double(1);double(1)]')  Remote=off
      settings: DataFormat=CANdb specified signals
  CAN Transmit1 : canlib/CAN Transmit  BlockHandle=2956.0023  DeviceMenu=Kvaser Virtual 1 (Channel 2)  Device=Kvaser Virtual 1 (Channel 2)  ObjConstructor=canChannel('Kvaser', 'Virtual 1', 2)  EnablePeriodicTransmit=off  MessagePeriod=1.000
  Ground9 : Ground
  Rate Transition : RateTransition
  Rate Transition1 : RateTransition
  wires:
  Bus Selector3/2 -> Rate Transition1/1  "<Inverter_Enable_Lockout>"
  Bus Selector3/1 -> Rate Transition/1  "<VSM_State>"
  Ground9/1 -> CAN Pack4/14, CAN Pack4/13, CAN Pack4/11, CAN Pack4/10, CAN Pack4/9, CAN Pack4/8, CAN Pack4/7, CAN Pack4/6, CAN Pack4/5, CAN Pack4/4, CAN Pack4/3, CAN Pack4/2
  EM/1 -> Bus Selector3/1
  Rate Transition/1 -> CAN Pack4/1
  Rate Transition1/1 -> CAN Pack4/12
  CAN Pack4/1 -> CAN Transmit1/1

== system EcoSIM3_P2_C2_WIP/Powertrain/Soft_ECUs_IO/VNT Kvaser/CANTx/EM/M171_Fault_Codes ==
  EM : Inport
  Bus Selector4 : BusSelector  OutputSignals=M171_Fault_Codes.POST_Fault,M171_Fault_Codes.RUN_Fault
  CAN Pack2 : canmsglib/CAN Pack  CANdbFile=C:\Users\EcoCAR_HIL\Documents\Khanna\EcoSIM3_P1_0_PHEV_TCU\Final_DBC\20150828 RMS PM CAN DB.dbc  MsgList=M171_Fault_Codes  MsgName=M171_Fault_Codes  MsgIDType=Standard (11-bit identifier)  MsgIdentifier=171  MsgLength=8  SignalInfo=D1_Post_Fault_Lo$0$16$1$2$1$0$1$0$0$65535$#D2_Post_Fault_Hi$16$16$1$2$1$0$1$0$0$65535$#D3_Run_Fault_Lo$32$16$1$2$1$0$1$0$0$65535$#D4_Run_Fault_Hi$48$16$1$2$1$0$1$0$0$65535$#  NSignals=4  StartBits=str2num('[int32(0);int32(16);int32(32);int32(48)]')  SignalSizes=str2num('[int32(16);int32(16);int32(16);int32(16)]')  ByteOrders=str2num('[int32(1);int32(1);int32(1);int32(1)]')  DataTypes=str2num('[int32(2);int32(2);int32(2);int32(2)]')  MultiplexTypes=str2num('[int32(1);int32(1);int32(1);int32(1)]')  MultiplexValues=str2num('[double(0);double(0);double(0);double(0)]')  Factors=str2num('[double(1);double(1);double(1);double(1)]')  Offsets=str2num('[double(0);double(0);double(0);double(0)]')  Minimums=str2num('[double(0);double(0);double(0);double(0)]')  Maximums=str2num('[double(65535);double(65535);double(65535);double(65535)]')  Remote=off
      settings: DataFormat=CANdb specified signals
  CAN Transmit1 : canlib/CAN Transmit  BlockHandle=2993.0023  DeviceMenu=Kvaser Virtual 1 (Channel 2)  Device=Kvaser Virtual 1 (Channel 2)  ObjConstructor=canChannel('Kvaser', 'Virtual 1', 2)  EnablePeriodicTransmit=off  MessagePeriod=1.000
  Ground2 : Ground
  Ground3 : Ground
  Rate Transition : RateTransition
  Rate Transition1 : RateTransition
  wires:
  Bus Selector4/2 -> Rate Transition1/1  "<RUN_Fault>"
  Bus Selector4/1 -> Rate Transition/1  "<POST_Fault>"
  Ground3/1 -> CAN Pack2/4
  Ground2/1 -> CAN Pack2/2
  EM/1 -> Bus Selector4/1
  Rate Transition/1 -> CAN Pack2/1
  Rate Transition1/1 -> CAN Pack2/3
  CAN Pack2/1 -> CAN Transmit1/1

== system EcoSIM3_P2_C2_WIP/Powertrain/Soft_ECUs_IO/VNT Kvaser/CANTx/EM/M172_Torque_And_Timer_Info ==
  EM : Inport
  Bus Selector2 : BusSelector  OutputSignals=M172_Torque_And_Timer_Info.EM_Torque_Out_Nm
  CAN Pack8 : canmsglib/CAN Pack  CANdbFile=C:\Users\EcoCAR_HIL\Documents\Khanna\EcoSIM3_P1_0_PHEV_TCU\Final_DBC\20150828 RMS PM CAN DB.dbc  MsgList=M172_Torque_And_Timer_Info  MsgName=M172_Torque_And_Timer_Info  MsgIDType=Standard (11-bit identifier)  MsgIdentifier=172  MsgLength=8  SignalInfo=D1_Commanded_Torque$0$16$1$1$1$0$1.000000e-01$0$-3.276800e+03$3.276700e+03$#D2_Torque_Feedback$16$16$1$1$1$0$1.000000e-01$0$-3.276800e+03$3.276700e+03$#D3_Power_On_Timer$32$32$1$2$1$0$3.000000e-03$0$0$4294970000$#  NSignals=3  StartBits=str2num('[int32(0);int32(16);int32(32)]')  SignalSizes=str2num('[int32(16);int32(16);int32(32)]')  ByteOrders=str2num('[int32(1);int32(1);int32(1)]')  DataTypes=str2num('[int32(1);int32(1);int32(2)]')  MultiplexTypes=str2num('[int32(1);int32(1);int32(1)]')  MultiplexValues=str2num('[double(0);double(0);double(0)]')  Factors=str2num('[double(1.000000e-01);double(1.000000e-01);double(3.000000e-03)]')  Offsets=str2num('[double(0);double(0);double(0)]')  Minimums=str2num('[double(-3.276800e+03);double(-3.276800e+03);double(0)]')  Maximums=str2num('[double(3.276700e+03);double(3.276700e+03);double(4294970000)]')  Remote=off
      settings: DataFormat=CANdb specified signals
  CAN Transmit1 : canlib/CAN Transmit  BlockHandle=3010.0023  DeviceMenu=Kvaser Virtual 1 (Channel 2)  Device=Kvaser Virtual 1 (Channel 2)  ObjConstructor=canChannel('Kvaser', 'Virtual 1', 2)  EnablePeriodicTransmit=off  MessagePeriod=1.000
  Ground4 : Ground
  Rate Transition : RateTransition
  wires:
  Bus Selector2/1 -> Rate Transition/1  "<EM_Torque_Out_Nm>"
  EM/1 -> Bus Selector2/1
  Ground4/1 -> CAN Pack8/1, CAN Pack8/3
  Rate Transition/1 -> CAN Pack8/2
  CAN Pack8/1 -> CAN Transmit1/1

== system EcoSIM3_P2_C2_WIP/Powertrain/Soft_ECUs_IO/VNT Kvaser/CANTx/ESS/BCM_Data ==
  ESS : Inport
  Bus Selector1 : BusSelector  OutputSignals=BCM_Data1.bcm_cell_tmax,BCM_Data1.bcm_cell_tmin,BCM_Data1.bcm_veh_mon
  CAN Pack6 : canmsglib/CAN Pack  CANdbFile=C:\Users\EcoCAR_HIL\Documents\Khanna\EcoSIM3_P1_0_PHEV_TCU\Final_DBC\BCM_VehBus_Std.dbc  MsgList=BCM_Data1  MsgName=BCM_Data1  MsgIDType=Standard (11-bit identifier)  MsgIdentifier=1072  MsgLength=8  SignalInfo=bcm_cell_tmax$32$8$2$2$1$0$5.000000e-01$-40$-40$85$#bcm_cell_tmin$40$8$2$2$1$0$5.000000e-01$-40$-40$85$#bcm_cell_vmax$8$13$2$2$1$0$1.000000e-03$0$0$5$#bcm_cell_vmin$24$13$2$2$1$0$1.000000e-03$0$0$5$#bcm_chga_ena$7$1$2$2$1$0$1$0$0$1$#bcm_chga_mon$22$1$2$2$1$0$1$0$0$1$#bcm_lvbat$56$8$2$2$1$0$1.000000e-01$0$0$25$#bcm_mod_ena$23$1$2$2$1$0$1$0$0$1$#bcm_veh_mon$21$1$2$2$1$0$1$0$0$1$#  NSignals=9  StartBits=str2num('[int32(32);int32(40);int32(8);int32(24);int32(7);int32(22);int32(56);int32(23);int32(21)]')  SignalSizes=str2num('[int32(8);int32(8);int32(13);int32(13);int32(1);int32(1);int32(8);int32(1);int32(1)]')  ByteOrders=str2num('[int32(2);int32(2);int32(2);int32(2);int32(2);int32(2);int32(2);int32(2);int32(2)]')  DataTypes=str2num('[int32(2);int32(2);int32(2);int32(2);int32(2);int32(2);int32(2);int32(2);int32(2)]')  MultiplexTypes=str2num('[int32(1);int32(1);int32(1);int32(1);int32(1);int32(1);int32(1);int32(1);int32(1)]')  MultiplexValues=str2num('[double(0);double(0);double(0);double(0);double(0);double(0);double(0);double(0);double(0)]')  Factors=str2num('[double(5.000000e-01);double(5.000000e-01);double(1.000000e-03);double(1.000000e-03);double(1);double(1);double(1.000000e-01);double(1);double(1)]')  Offsets=str2num('[double(-40);double(-40);double(0);double(0);double(0);double(0);double(0);double(0);double(0)]')  Minimums=str2num('[double(-40);double(-40);double(0);double(0);double(0);double(0);double(0);double(0);double(0)]')  Maximums=str2num('[double(85);double(85);double(5);double(5);double(1);double(1);double(25);double(1);double(1)]')  Remote=off
      settings: DataFormat=CANdb specified signals
  CAN Transmit6 : canlib/CAN Transmit  BlockHandle=3038.0023  DeviceMenu=Kvaser Virtual 1 (Channel 1)  Device=Kvaser Virtual 1 (Channel 1)  ObjConstructor=canChannel('Kvaser', 'Virtual 1', 1)  EnablePeriodicTransmit=off  MessagePeriod=1.000
  Ground{14..19} (6 alike) : Ground
  Rate Transition : RateTransition
  Rate Transition1 : RateTransition
  Rate Transition2 : RateTransition
  wires:
  Ground15/1 -> CAN Pack6/4
  Bus Selector1/2 -> Rate Transition1/1  "<bcm_cell_tmin>"
  Ground16/1 -> CAN Pack6/5
  Ground19/1 -> CAN Pack6/8
  Ground17/1 -> CAN Pack6/6
  Ground18/1 -> CAN Pack6/7
  Ground14/1 -> CAN Pack6/3
  Bus Selector1/3 -> Rate Transition2/1  "<bcm_veh_mon>"
  Bus Selector1/1 -> Rate Transition/1  "<bcm_cell_tmax>"
  ESS/1 -> Bus Selector1/1
  Rate Transition/1 -> CAN Pack6/1
  Rate Transition1/1 -> CAN Pack6/2
  Rate Transition2/1 -> CAN Pack6/9
  CAN Pack6/1 -> CAN Transmit6/1

== system EcoSIM3_P2_C2_WIP/Powertrain/Soft_ECUs_IO/VNT Kvaser/CANTx/ESS/BCM_Limits ==
  ESS : Inport
  Bus Selector1 : BusSelector  OutputSignals=BCM_Limits.bcm_chg_buf,BCM_Limits.bcm_dis_buf
  CAN Pack1 : canmsglib/CAN Pack  CANdbFile=C:\Users\EcoCAR_HIL\Documents\Khanna\EcoSIM3_P1_0_PHEV_TCU\Final_DBC\BCM_VehBus_Std.dbc  MsgList=BCM_Limits  MsgName=BCM_Limits  MsgIDType=Standard (11-bit identifier)  MsgIdentifier=1056  MsgLength=8  SignalInfo=bcm_cell_overvolt$55$1$2$2$1$0$1$0$0$1$#bcm_cell_undervolt$54$1$2$2$1$0$1$0$0$1$#bcm_chg_buf$32$8$2$2$1$0$5.000000e-01$0$0$100$#bcm_chg_max$16$12$2$2$1$0$2.500000e-01$0$0$1000$#bcm_dis_buf$24$8$2$2$1$0$5.000000e-01$0$0$100$#bcm_dis_max$12$12$2$2$1$0$2.500000e-01$0$0$1000$#bcm_t_coolant$40$8$2$2$1$0$5.000000e-01$-40$-40$85$#  NSignals=7  StartBits=str2num('[int32(55);int32(54);int32(32);int32(16);int32(24);int32(12);int32(40)]')  SignalSizes=str2num('[int32(1);int32(1);int32(8);int32(12);int32(8);int32(12);int32(8)]')  ByteOrders=str2num('[int32(2);int32(2);int32(2);int32(2);int32(2);int32(2);int32(2)]')  DataTypes=str2num('[int32(2);int32(2);int32(2);int32(2);int32(2);int32(2);int32(2)]')  MultiplexTypes=str2num('[int32(1);int32(1);int32(1);int32(1);int32(1);int32(1);int32(1)]')  MultiplexValues=str2num('[double(0);double(0);double(0);double(0);double(0);double(0);double(0)]')  Factors=str2num('[double(1);double(1);double(5.000000e-01);double(2.500000e-01);double(5.000000e-01);double(2.500000e-01);double(5.000000e-01)]')  Offsets=str2num('[double(0);double(0);double(0);double(0);double(0);double(0);double(-40)]')  Minimums=str2num('[double(0);double(0);double(0);double(0);double(0);double(0);double(-40)]')  Maximums=str2num('[double(1);double(1);double(100);double(1000);double(100);double(1000);double(85)]')  Remote=off
      settings: DataFormat=CANdb specified signals
  CAN Transmit6 : canlib/CAN Transmit  BlockHandle=3066.0023  DeviceMenu=Kvaser Virtual 1 (Channel 1)  Device=Kvaser Virtual 1 (Channel 1)  ObjConstructor=canChannel('Kvaser', 'Virtual 1', 1)  EnablePeriodicTransmit=off  MessagePeriod=1.000
  Ground{4,6..9} (5 alike) : Ground
  Rate Transition : RateTransition
  Rate Transition1 : RateTransition
  wires:
  Ground8/1 -> CAN Pack1/6
  Ground4/1 -> CAN Pack1/1
  Ground9/1 -> CAN Pack1/7
  Ground7/1 -> CAN Pack1/4
  Ground6/1 -> CAN Pack1/2
  Bus Selector1/1 -> Rate Transition/1  "<bcm_chg_buf>"
  ESS/1 -> Bus Selector1/1
  Bus Selector1/2 -> Rate Transition1/1  "<bcm_dis_buf>"
  Rate Transition/1 -> CAN Pack1/3
  Rate Transition1/1 -> CAN Pack1/5
  CAN Pack1/1 -> CAN Transmit6/1

== system EcoSIM3_P2_C2_WIP/Powertrain/Soft_ECUs_IO/VNT Kvaser/CANTx/ESS/BCM_Status ==
  ESS : Inport
  Bus Selector3 : BusSelector  OutputSignals=BCM_Status.bcm_chgc_stat,BCM_Status.bcm_cpwr_cmd,BCM_Status.bcm_cpwr_mon,BCM_Status.bcm_epo,BCM_Status.bcm_hvil_mon,BCM_Status.bcm_ibat,BCM_Status.bcm_mainc_stat,BCM_Status.bcm_on_plug,BCM_Status.bcm_ready,BCM_Status.bcm_soc,BCM_Status.bcm_vbat
  CAN Pack2 : canmsglib/CAN Pack  CANdbFile=C:\Users\EcoCAR_HIL\Documents\Khanna\EcoSIM3_P1_0_PHEV_TCU\Final_DBC\BCM_VehBus_Std.dbc  MsgList=BCM_Status  MsgName=BCM_Status  MsgIDType=Standard (11-bit identifier)  MsgIdentifier=1040  MsgLength=8  SignalInfo=bcm_alarm$14$2$2$2$1$0$1$0$0$3$#bcm_chg_done$52$1$2$2$1$0$1$0$0$1$#bcm_chgc_stat$6$2$2$2$1$0$1$0$0$2$#bcm_cool_req$53$1$2$2$1$0$1$0$0$1$#bcm_cpwr_cmd$12$1$2$2$1$0$1$0$0$1$#bcm_cpwr_mon$13$1$2$2$1$0$1$0$0$1$#bcm_epo$1$1$2$2$1$0$1$0$0$1$#bcm_gfd$16$12$2$2$1$0$2.500000e-01$0$0$1000$#bcm_hvil_mon$3$1$2$2$1$0$1$0$0$1$#bcm_ibat$40$16$2$2$1$0$2.500000e-02$-1000$-1000$500$#bcm_lls_status$54$2$2$2$1$0$1$0$0$3$#bcm_mainc_stat$4$2$2$2$1$0$1$0$0$2$#bcm_on_plug$2$1$2$2$1$0$1$0$0$1$#bcm_ready$0$1$2$2$1$0$1$0$0$1$#bcm_soc$24$8$2$2$1$0$5.000000e-01$0$0$100$#bcm_vbat$56$12$2$2$1$0$2.500000e-01$0$0$1000$#  NSignals=16  StartBits=str2num('[int32(14);int32(52);int32(6);int32(53);int32(12);int32(13);int32(1);int32(16);int32(3);int32(40);int32(54);int32(4);int32(2);int32(0);int32(24);int32(56)]')  SignalSizes=str2num('[int32(2);int32(1);int32(2);int32(1);int32(1);int32(1);int32(1);int32(12);int32(1);int32(16);int32(2);int32(2);int32(1);int32(1);int32(8);int32(12)]')  ByteOrders=str2num('[int32(2);int32(2);int32(2);int32(2);int32(2);int32(2);int32(2);int32(2);int32(2);int32(2);int32(2);int32(2);int32(2);int32(2);int32(2);int32(2)]')  DataTypes=str2num('[int32(2);int32(2);int32(2);int32(2);int32(2);int32(2);int32(2);int32(2);int32(2);int32(2);int32(2);int32(2);int32(2);int32(2);int32(2);int32(2)]')  MultiplexTypes=str2num('[int32(1);int32(1);int32(1);int32(1);int32(1);int32(1);int32(1);int32(1);int32(1);int32(1);int32(1);int32(1);int32(1);int32(1);int32(1);int32(1)]')  MultiplexValues=str2num('[double(0);double(0);double(0);double(0);double(0);double(0);double(0);double(0);double(0);double(0);double(0);double(0);double(0);double(0);double(0);double(0)]')  Factors=str2num('[double(1);double(1);double(1);double(1);double(1);double(1);double(1);double(2.500000e-01);double(1);double(2.500000e-02);double(1);double(1);double(1);double(1);double(5.000000e-01);double(2.500000e-01)]')  Offsets=str2num('[double(0);double(0);double(0);double(0);double(0);double(0);double(0);double(0);double(0);double(-1000);double(0);double(0);double(0);double(0);double(0);double(0)]')  Minimums=str2num('[double(0);double(0);double(0);double(0);double(0);double(0);double(0);double(0);double(0);double(-1000);double(0);double(0);double(0);double(0);double(0);double(0)]')  Maximums=str2num('[double(3);double(1);double(2);double(1);double(1);double(1);double(1);double(1000);double(1);double(500);double(3);double(2);double(1);double(1);double(100);double(1000)]')  Remote=off
      settings: DataFormat=CANdb specified signals
  CAN Transmit6 : canlib/CAN Transmit  BlockHandle=3089.0018  DeviceMenu=Kvaser Virtual 1 (Channel 1)  Device=Kvaser Virtual 1 (Channel 1)  ObjConstructor=canChannel('Kvaser', 'Virtual 1', 1)  EnablePeriodicTransmit=off  MessagePeriod=1.000
  Ground{,1..3,5} (5 alike) : Ground
  Rate Transition : RateTransition
  Rate Transition10 : RateTransition  Deterministic=off
  Rate Transition11 : RateTransition  Deterministic=off
  Rate Transition9 : RateTransition  Deterministic=off
  Scope : Scope
      settings: SaveName=ScopeData13
  wires:
  Rate Transition10/1 -> CAN Pack2/10
  Rate Transition9/1 -> CAN Pack2/16
  Ground/1 -> CAN Pack2/1
  Ground1/1 -> CAN Pack2/2
  Rate Transition11/1 -> CAN Pack2/15
  Ground3/1 -> CAN Pack2/8
  Ground2/1 -> CAN Pack2/4
  Ground5/1 -> CAN Pack2/11
  Bus Selector3/2 -> CAN Pack2/5  "<bcm_cpwr_cmd>"
  Bus Selector3/3 -> CAN Pack2/6  "<bcm_cpwr_mon>"
  Bus Selector3/1 -> Rate Transition/1  "<bcm_chgc_stat>"
  ESS/1 -> Bus Selector3/1
  Bus Selector3/4 -> CAN Pack2/7  "<bcm_epo>"
  Bus Selector3/5 -> CAN Pack2/9  "<bcm_hvil_mon>"
  Bus Selector3/7 -> Scope/1, CAN Pack2/12  "<bcm_mainc_stat>"
  Bus Selector3/6 -> Rate Transition10/1  "<bcm_ibat>"
  Bus Selector3/8 -> CAN Pack2/13  "<bcm_on_plug>"
  Bus Selector3/9 -> CAN Pack2/14  "<bcm_ready>"
  Bus Selector3/10 -> Rate Transition11/1  "<bcm_soc>"
  Bus Selector3/11 -> Rate Transition9/1  "<bcm_vbat>"
  Rate Transition/1 -> CAN Pack2/3
  CAN Pack2/1 -> CAN Transmit6/1
